simulink model "modello_completo_simulink2020"  (R2020a)
settings: Solver=VariableStepAuto  StartTime=0.0  StopTime=200  RelTol=1e-3
values from neighbouring files (symbols this model uses):
  a = 0.35    [data.m]    (also in geodetic2nedS.m = 6378137)
  a1 = rho * D^4 * alpha1    (= 0.000388302366464)    [data.m]
  a2 = -rho * D^3 * alpha2 * (1 - omega)    (= 0.0037030698432)    [data.m]
  AHRS_bias = [0 0 0]    [data.m]
  AHRS_sample_time = 1/50    (= 0.02)    [data.m]
  AHRS_var = ([1 1 2] * pi/180).^2    [data.m]
  alpha1 = 0.0113    [data.m]
  alpha2 = -0.0091    [data.m]
  c = son2(1)    [Sonar_id.m]    (also in data.m = 0.19)
  current = [seaCurrent; 0; 0; 0]    [data.m]
  D = 0.076    [data.m]
  dead_zone_limit = 31.5    [data.m]
  DVL_sample_t = 1/12    (= 0.0833333333333)    [data.m]
  DVL_var1 = 0.005^2    (= 2.5e-05)    [data.m]
  DVL_var2 = 0.015^2    (= 0.000225)    [data.m]
  DVL_var3 = 0.023^2    (= 0.000529)    [data.m]
  gps_sample_t = 1    [data.m]
  H = eye(3)    [data.m]    (also in navigation_data.m)
  IMU_sample_time = 1/100    (= 0.01)    [data.m]
  initial = []    [data.m]
  INSP = unicode2native(inspectionDirection)    [data.m]
  Ki_bodypos1 = 0    [parametri_PID.m]
  Ki_bodypos2 = 0    [parametri_PID.m]
  Ki_bodypos3 = 0    [parametri_PID.m]
  Ki_bodypos4 = 0    [parametri_PID.m]
  Ki_bodypos5 = 0    [parametri_PID.m]
  Ki_depth1 = 0    [parametri_PID.m]
  Ki_depth2 = 0    [parametri_PID.m]
  Ki_depth3 = 0    [parametri_PID.m]
  Ki_depth4 = 0    [parametri_PID.m]
  Ki_depth5 = 0    [parametri_PID.m]
  Ki_latvel1 = 0    [parametri_PID.m]
  Ki_latvel2 = 0    [parametri_PID.m]
  Ki_latvel3 = 0    [parametri_PID.m]
  Ki_latvel4 = 0    [parametri_PID.m]
  Ki_latvel5 = 0    [parametri_PID.m]
  Ki_P1 = 0    [parametri_PID.m]
  Ki_P2 = 0    [parametri_PID.m]
  Ki_P3 = 0    [parametri_PID.m]
  Ki_P4 = 0    [parametri_PID.m]
  Ki_P5 = 0    [parametri_PID.m]
  Ki_R1 = 0    [parametri_PID.m]
  Ki_R2 = 0    [parametri_PID.m]
  Ki_R3 = 0    [parametri_PID.m]
  Ki_R4 = 0    [parametri_PID.m]
  Ki_R5 = 0    [parametri_PID.m]
  Ki_rel_or1 = 0    [parametri_PID.m]
  Ki_rel_or2 = 0    [parametri_PID.m]
  Ki_rel_or3 = 0    [parametri_PID.m]
  Ki_rel_or4 = 0    [parametri_PID.m]
  Ki_rel_or5 = 0    [parametri_PID.m]
  Ki_reldist1 = 0    [parametri_PID.m]
  Ki_reldist2 = 0    [parametri_PID.m]
  Ki_reldist3 = 0    [parametri_PID.m]
  Ki_reldist4 = 0    [parametri_PID.m]
  Ki_reldist5 = 0    [parametri_PID.m]
  Ki_surge1 = 0    [parametri_PID.m]
  Ki_surge2 = 0    [parametri_PID.m]
  Ki_surge3 = 0    [parametri_PID.m]
  Ki_surge4 = 0    [parametri_PID.m]
  Ki_surge5 = 0    [parametri_PID.m]
  Ki_yaw1 = 0    [parametri_PID.m]
  Ki_yaw2 = 0    [parametri_PID.m]
  Ki_yaw3 = 0    [parametri_PID.m]
  Ki_yaw4 = 0    [parametri_PID.m]
  Ki_yaw5 = 0    [parametri_PID.m]
  Kp_bodypos1 = 0    [parametri_PID.m]
  Kp_bodypos2 = 2    [parametri_PID.m]
  Kp_bodypos3 = 2    [parametri_PID.m]
  Kp_bodypos4 = 2    [parametri_PID.m]
  Kp_bodypos5 = 2    [parametri_PID.m]
  Kp_depth1 = 0    [parametri_PID.m]
  Kp_depth2 = 2    [parametri_PID.m]
  Kp_depth3 = 2    [parametri_PID.m]
  Kp_depth4 = 2    [parametri_PID.m]
  Kp_depth5 = 2    [parametri_PID.m]
  Kp_latvel1 = 0    [parametri_PID.m]
  Kp_latvel2 = 2    [parametri_PID.m]
  Kp_latvel3 = 2    [parametri_PID.m]
  Kp_latvel4 = 2    [parametri_PID.m]
  Kp_latvel5 = 2    [parametri_PID.m]
  Kp_P1 = 0    [parametri_PID.m]
  Kp_P2 = 2    [parametri_PID.m]
  Kp_P3 = 2    [parametri_PID.m]
  Kp_P4 = 2    [parametri_PID.m]
  Kp_P5 = 2    [parametri_PID.m]
  Kp_R1 = 0    [parametri_PID.m]
  Kp_R2 = 2    [parametri_PID.m]
  Kp_R3 = 2    [parametri_PID.m]
  Kp_R4 = 2    [parametri_PID.m]
  Kp_R5 = 2    [parametri_PID.m]
  Kp_rel_or1 = 0    [parametri_PID.m]
  Kp_rel_or2 = 2    [parametri_PID.m]
  Kp_rel_or3 = 2    [parametri_PID.m]
  Kp_rel_or4 = 2    [parametri_PID.m]
  Kp_rel_or5 = 2    [parametri_PID.m]
  Kp_reldist1 = 0    [parametri_PID.m]
  Kp_reldist2 = 2    [parametri_PID.m]
  Kp_reldist3 = 2    [parametri_PID.m]
  Kp_reldist4 = 2    [parametri_PID.m]
  Kp_reldist5 = 2    [parametri_PID.m]
  Kp_surge1 = 0    [parametri_PID.m]
  Kp_surge2 = 2    [parametri_PID.m]
  Kp_surge3 = 2    [parametri_PID.m]
  Kp_surge4 = 2    [parametri_PID.m]
  Kp_surge5 = 2    [parametri_PID.m]
  Kp_yaw1 = 0.6*6    (= 3.6)    [parametri_PID.m]
  Kp_yaw2 = 2    [parametri_PID.m]
  Kp_yaw3 = 2    [parametri_PID.m]
  Kp_yaw4 = 2    [parametri_PID.m]
  Kp_yaw5 = 2    [parametri_PID.m]
  M = M_rb + M_a    [Masse.m]
  M_inv = inv(M)    [Masse.m]
  n_max = 340    [data.m]
  num_cycle = 5    [data.m]    (also in navigation_data.m)
  omega = 0.1    [data.m]
  plot_smpl = 0.1    [data.m]
  ps_sample_t = 0.02    [data.m]
  ps_var = (5000/3)^2    (= 2777777.77778)    [data.m]
  pylonCenter = [ 43.723046 ... (first row only)    [missionB.m]
  ... (+4 more)
undefined symbols (not defined in the file or in its folder): DiscIntNeverNeededParam, s_data
libraries: simulink x3
(part 2 of 5)

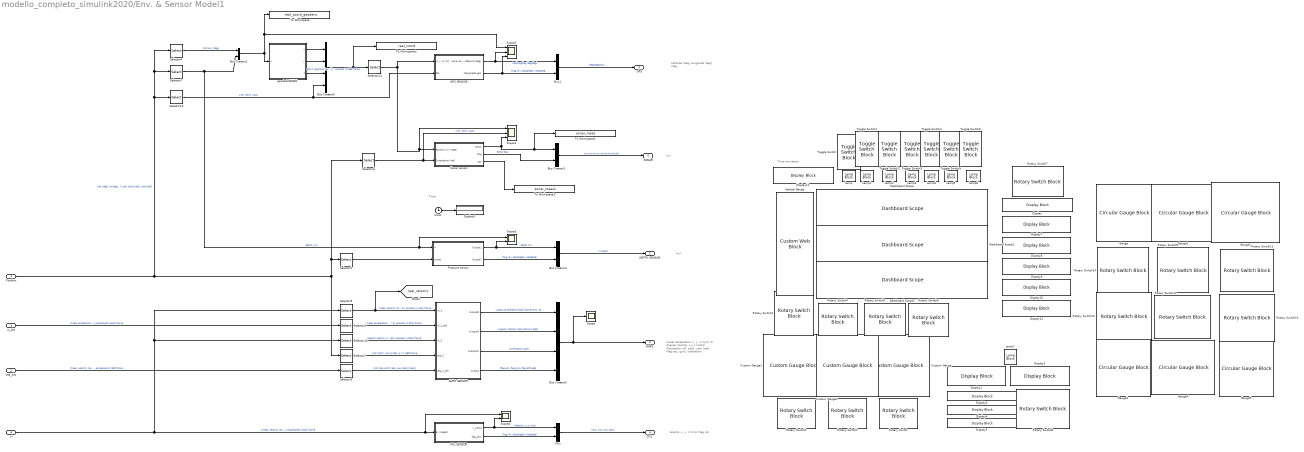
== system modello_completo_simulink2020/Env. & Sensor Model1 ==
  note: Time simulation
  note: Time
  note: (m)
  note: Velocity x, y, z (m/s)
      | Flag dvl
  note: Linear Acceleration x, y, z (m/s^2)
      | Angular Velocity x,y,z (rad/s)
      | Orientation roll, pitch, yaw (rad)
      | Flag acc, gyro, orientation
  note: (m)
  note: Latitude (deg)
      | Longitude (deg)
      | Flag
  Position : Inport
  eta_dot : Inport  Port=2
  ni_dot : Inport  Port=3
  ni : Inport  Port=4
  AHRS SENSOR : Subsystem
  Bus Creator2 : BusCreator  Inputs=2
  Bus Creator3 : BusCreator  Inputs=2
  Bus Creator4 : BusCreator  Inputs=2
  Bus Creator5 : BusCreator  Inputs=4
  Bus Creator6 : BusCreator  Inputs=4
  Clock : Clock
  Custom Gauge : CustomGaugeBlock  LabelPosition=Bottom  NeedleImage=data:image/svg+xml;base64,PD94bWwgdmVyc2lvbj0iMS4wIiBlbmNvZGluZz0idXRmLTgiPz4KPCEtLSBHZW5lcmF0b3I6IEFkb2JlIElsbHVzdHJhdG9yIDE5LjIuMSwgU1ZHIEV4cG9ydCBQbHVnLUluIC4gU1ZHIFZlcnNpb246IDYuMDAgQnVpbGQgMCkgIC0tPgo8c3ZnIHZlcnNpb249IjEuMSIgeG1sbnM9Imh0dHA6Ly93d3cudzMub3JnLzIwMDAvc3ZnIiB4bWxuczp4bGluaz0iaHR0cDovL3d3dy53My5vcmcvMTk5OS94bGluayIgeD0iMHB4IiB5PSIwcHgiCgkgdmlld0JveD0iMCAwIDIwMCA1MCIgc3R5bGU9ImVuYWJsZS1iYWNrZ3JvdW5kOm5ldyAw ...(+9940 chars)  NeedleXPos=0.4166541406625117  NeedleYPos=0.48689867826277666  NeedleHeight=0.08073723570250356  NeedleWidth=0.1330086340281622  NeedleInitialRotation=-59.94322499147643  BackgroundImage=data:image/svg+xml;base64,PD94bWwgdmVyc2lvbj0iMS4wIiBlbmNvZGluZz0iVVRGLTgiIHN0YW5kYWxvbmU9Im5vIj8+CjwhLS0gR2VuZXJhdG9yOiBBZG9iZSBJbGx1c3RyYXRvciAxOS4yLjEsIFNWRyBFeHBvcnQgUGx1Zy1JbiAuIFNWRyBWZXJzaW9uOiA2LjAwIEJ1aWxkIDApICAtLT4KCjxzdmcKICAgeG1sbnM6ZGM9Imh0dHA6Ly9wdXJsLm9yZy9kYy9lbGVtZW50cy8xLjEvIgogICB4bWxuczpjYz0iaHR0cDovL2NyZWF0aXZlY29tbW9ucy5vcmcvbnMjIgogICB4bWxuczpyZGY9Imh0dHA6Ly93d3cudzMub3JnLzE5OTkvMDIvMjItcmRmLXN5bnRh ...(+9660 chars)  GaugeMin=-1  GaugeMax=1  GaugeArcDefined=true  GaugeArcRadius=0.09453995649289303  GaugeArcStrokeWidth=0.027647132727189508  GaugeArcRotation=240.5385250290321  GaugeArcRatio=0.8333333333333  GaugeArcTransparency=0  ValueArcColor=#1759b0  GaugeTickColor=#faf5c8  ScaleColorsJSON=[]  fixedAspectRatio=on  IsLinearGauge=false  GaugeTrackLeft=0.35  GaugeTrackTop=0.35  GaugeTrackHeight=0.1  GaugeTrackWidth=0.3  GaugeTrackRotation=0  ScaleMin=-1
  Custom Gauge1 : CustomGaugeBlock  LabelPosition=Bottom  NeedleImage=data:image/svg+xml;base64,PD94bWwgdmVyc2lvbj0iMS4wIiBlbmNvZGluZz0idXRmLTgiPz4KPCEtLSBHZW5lcmF0b3I6IEFkb2JlIElsbHVzdHJhdG9yIDE5LjIuMSwgU1ZHIEV4cG9ydCBQbHVnLUluIC4gU1ZHIFZlcnNpb246IDYuMDAgQnVpbGQgMCkgIC0tPgo8c3ZnIHZlcnNpb249IjEuMSIgeG1sbnM9Imh0dHA6Ly93d3cudzMub3JnLzIwMDAvc3ZnIiB4bWxuczp4bGluaz0iaHR0cDovL3d3dy53My5vcmcvMTk5OS94bGluayIgeD0iMHB4IiB5PSIwcHgiCgkgdmlld0JveD0iMCAwIDIwMCA1MCIgc3R5bGU9ImVuYWJsZS1iYWNrZ3JvdW5kOm5ldyAw ...(+9940 chars)  NeedleXPos=0.4141461298017858  NeedleYPos=0.4865044384352907  NeedleHeight=0.08316674888547909  NeedleWidth=0.13701107759722064  NeedleInitialRotation=-59.94322499147643  BackgroundImage=data:image/svg+xml;base64,PD94bWwgdmVyc2lvbj0iMS4wIiBlbmNvZGluZz0iVVRGLTgiIHN0YW5kYWxvbmU9Im5vIj8+CjwhLS0gR2VuZXJhdG9yOiBBZG9iZSBJbGx1c3RyYXRvciAxOS4yLjEsIFNWRyBFeHBvcnQgUGx1Zy1JbiAuIFNWRyBWZXJzaW9uOiA2LjAwIEJ1aWxkIDApICAtLT4KCjxzdmcKICAgeG1sbnM6ZGM9Imh0dHA6Ly9wdXJsLm9yZy9kYy9lbGVtZW50cy8xLjEvIgogICB4bWxuczpjYz0iaHR0cDovL2NyZWF0aXZlY29tbW9ucy5vcmcvbnMjIgogICB4bWxuczpyZGY9Imh0dHA6Ly93d3cudzMub3JnLzE5OTkvMDIvMjItcmRmLXN5bnRh ...(+9660 chars)  GaugeMin=-1  GaugeMax=1  GaugeArcDefined=true  GaugeArcRadius=0.09738481572815044  GaugeArcStrokeWidth=0.028479079385354485  GaugeArcRotation=240.5385250290321  GaugeArcRatio=0.8333333333333  GaugeArcTransparency=0  ValueArcColor=#1759b0  GaugeTickColor=#faf5c8  ScaleColorsJSON=[]  fixedAspectRatio=on  IsLinearGauge=false  GaugeTrackLeft=0.35  GaugeTrackTop=0.35  GaugeTrackHeight=0.1  GaugeTrackWidth=0.3  GaugeTrackRotation=0  ScaleMin=-1
  Custom Gauge2 : CustomGaugeBlock  LabelPosition=Bottom  NeedleImage=data:image/svg+xml;base64,PD94bWwgdmVyc2lvbj0iMS4wIiBlbmNvZGluZz0idXRmLTgiPz4KPCEtLSBHZW5lcmF0b3I6IEFkb2JlIElsbHVzdHJhdG9yIDE5LjIuMSwgU1ZHIEV4cG9ydCBQbHVnLUluIC4gU1ZHIFZlcnNpb246IDYuMDAgQnVpbGQgMCkgIC0tPgo8c3ZnIHZlcnNpb249IjEuMSIgeG1sbnM9Imh0dHA6Ly93d3cudzMub3JnLzIwMDAvc3ZnIiB4bWxuczp4bGluaz0iaHR0cDovL3d3dy53My5vcmcvMTk5OS94bGluayIgeD0iMHB4IiB5PSIwcHgiCgkgdmlld0JveD0iMCAwIDIwMCA1MCIgc3R5bGU9ImVuYWJsZS1iYWNrZ3JvdW5kOm5ldyAw ...(+9940 chars)  NeedleXPos=0.4166541406625117  NeedleYPos=0.48689867826277666  NeedleHeight=0.08073723570250356  NeedleWidth=0.1330086340281622  NeedleInitialRotation=-59.94322499147643  BackgroundImage=data:image/svg+xml;base64,PD94bWwgdmVyc2lvbj0iMS4wIiBlbmNvZGluZz0iVVRGLTgiIHN0YW5kYWxvbmU9Im5vIj8+CjwhLS0gR2VuZXJhdG9yOiBBZG9iZSBJbGx1c3RyYXRvciAxOS4yLjEsIFNWRyBFeHBvcnQgUGx1Zy1JbiAuIFNWRyBWZXJzaW9uOiA2LjAwIEJ1aWxkIDApICAtLT4KCjxzdmcKICAgeG1sbnM6ZGM9Imh0dHA6Ly9wdXJsLm9yZy9kYy9lbGVtZW50cy8xLjEvIgogICB4bWxuczpjYz0iaHR0cDovL2NyZWF0aXZlY29tbW9ucy5vcmcvbnMjIgogICB4bWxuczpyZGY9Imh0dHA6Ly93d3cudzMub3JnLzE5OTkvMDIvMjItcmRmLXN5bnRh ...(+9660 chars)  GaugeMin=-1  GaugeMax=1  GaugeArcDefined=true  GaugeArcRadius=0.09453995649289303  GaugeArcStrokeWidth=0.027647132727189508  GaugeArcRotation=240.5385250290321  GaugeArcRatio=0.8333333333333  GaugeArcTransparency=0  ValueArcColor=#1759b0  GaugeTickColor=#faf5c8  ScaleColorsJSON=[]  fixedAspectRatio=on  IsLinearGauge=false  GaugeTrackLeft=0.35  GaugeTrackTop=0.35  GaugeTrackHeight=0.1  GaugeTrackWidth=0.3  GaugeTrackRotation=0  ScaleMin=-1
  DVL SENSOR : Subsystem
  Dashboard Scope : DashboardScope  Ymin=-12  Ymax=12  LegendPosition=Right
  Dashboard Scope1 : DashboardScope  Ymin=-1  Ymax=1  LegendPosition=Right
  Dashboard Scope2 : DashboardScope  Ymin=-2  Ymax=2  LegendPosition=Right
  Display : DisplayBlock  LabelPosition=Hide  Format=Custom  Transparency=1  FormatString=Sonar flag: %d %d %d %d %d
  Display1 : DisplayBlock  LabelPosition=Hide  Format=Custom  Transparency=1  FormatString=Lat: %f °
  Display{8..11} (4 alike) : DisplayBlock  Format=short  Transparency=1
  Display12 : DisplayBlock  LabelPosition=Hide  Format=Custom  Transparency=1  FormatString=%.1f s
  Display2 : DisplayBlock  LabelPosition=Hide  Format=Custom  Transparency=1  FormatString=Lon: %f °
  Display3 : DisplayBlock  LabelPosition=Hide  Format=Custom  Transparency=1  FormatString=X NED: %.3f m
  Display4 : DisplayBlock  LabelPosition=Hide  Format=Custom  Transparency=1  FormatString=Y NED: %.3f m
  Display5 : DisplayBlock  LabelPosition=Hide  Format=Custom  Transparency=1  FormatString=Z NED: %.3f m
  Display6 : Display
  Display7 : DisplayBlock  Format=short  Transparency=1  FormatString=%d m
  GPS SENSOR : Subsystem
  Gauge : CircularGaugeBlock  ScaleMin=-25  ScaleMax=25
  Gauge1 : CircularGaugeBlock  ScaleMin=-25  ScaleMax=25
  Gauge2 : CircularGaugeBlock  ScaleMin=-25  ScaleMax=25
  Gauge3 : CircularGaugeBlock  LabelPosition=Bottom  ScaleMin=-45  ScaleMax=45
  Gauge4 : CircularGaugeBlock  LabelPosition=Bottom  ScaleMin=-45  ScaleMax=45
  Gauge5 : CircularGaugeBlock  LabelPosition=Bottom  ScaleMin=-45  ScaleMax=45
  Lamp{,1..7} (8 alike) : LampBlock  LabelPosition=Hide
  Mux : Mux  Inputs=2
  Mux1 : Mux  Inputs=2
  Pressure sensor : Subsystem
  Rotary Switch{,1..8} (9 alike) : RotarySwitchBlock  LabelPosition=Bottom
      settings: Values={{'Off', 'On', '50%', '200%'}, [0 1 0.5 2]}
  Rotary Switch{9..14} (6 alike) : RotarySwitchBlock
  Scope : Scope
  Scope1 : Scope  NumInputPorts=3
  Scope2 : Scope  NumInputPorts=3
  Scope3 : Scope  NumInputPorts=2
  Scope4 : Scope  NumInputPorts=2
  Selector{1..3,6,10,12} (6 alike) : Selector  InputPortWidth=6  IndexOptions=Index vector (dialog)  Indices=[4 5 6]  OutputSizes=1
  Selector14 : Selector  InputPortWidth=6  IndexOptions=Index vector (dialog)  Indices=[1 2 3]  OutputSizes=1
  Selector4 : Selector  InputPortWidth=6  IndexOptions=Index vector (dialog)  Indices=[1 2]  OutputSizes=1
  Selector5 : Selector  InputPortWidth=6  IndexOptions=Index vector (dialog)  Indices=[1 2 3]  OutputSizes=1
  Selector7 : Selector  InputPortWidth=6  IndexOptions=Index vector (dialog)  Indices=[3]  OutputSizes=1
  Selector9 : Selector  InputPortWidth=6  IndexOptions=Index vector (dialog)  Indices=[1 2 3]  OutputSizes=1
  Sonar sensor : Subsystem
  To Workspace : ToWorkspace  VariableName=real_coord_geodetic  SampleTime=-1
  To Workspace1 : ToWorkspace  VariableName=sonar_meas  SampleTime=plot_smpl
  To Workspace2 : ToWorkspace  VariableName=real_coord  SampleTime=plot_smpl
  To Workspace3 : ToWorkspace  VariableName=sonar_meas1  SampleTime=plot_smpl
  Toggle Switch{,2,4,6} (4 alike) : ToggleSwitchBlock  LabelPosition=Bottom
      settings: Values={{'Off', 'On'}, [0 1]}
  Toggle Switch1 : ToggleSwitchBlock
      settings: Values={{'Off', 'On'}, [1 0]}
  Toggle Switch3 : ToggleSwitchBlock
      settings: Values={{'Off', 'On'}, [0 1]}
  Toggle Switch5 : ToggleSwitchBlock
      settings: Values={{'Off', 'On'}, [0 1]}
  Vertical Gauge : CustomWebBlock  ShowInitialText=on  Configuration="{\"components\":[{\"name\":\"LinearScaleComponent\",\"settings\":{\"bounds\":{\"max\":40,\"min\":0,\"tickInterval\":\"auto\"},\"labelColor\":[250,245,199],\"labelFont\":{\"font\":\"Arial\",\"fontSize\":12},\"labelTransparency\":1,\"needleImage\":{\"size\":[21,75],\"src\":\"data:image\\/svg+xml;base64,PHN2ZyB4bWxucz0iaHR0cDovL3d3dy53My5vcmcvMjAwMC9zdmciIHhtbG5zOnhsaW5rPSJodHRwOi8vd3d3LnczLm9yZy8xOTk5L3hsaW5rIiB2aWV3Qm94PSIwIDAgMjEgNzUiPjxkZWZzPjxzdHlsZT4uY2xzLTF7ZmlsbDpub25lO30uY2xzLTJ7aXNvbGF0aW9uOmlzb2xhdGU7fS5jbHMtM3tjbGlwLXBhdGg6dXJsKCNjbGlwLXBhdGgpO30uY2xzLTR7b3BhY2l0eTowLjM7bWl4LWJsZW5kLW1vZGU6bXVsdGlwbHk7fS5jbHMtNXtmaWxsOiNlYjI2Mjk7fTwvc3R5bGU+PGNsaXBQYXRoIGlkPSJjbGlwLXBhdGgiIHRyYW5zZm9y ...(+1928 chars)\",\"srcOrientation\":\"horizontal\"},\"needleOffset\":[-0.01094391244870041,0],\"needleSize\":{\"height\":0.11960078534031414,\"width\":0.7589285714285714},\"position\":[0.015887605042016806,0.06986607142857143,0.8,0.9641544117647058],\"scaleColorSize\":0.24,\"scaleColors\":[],\"scaleColorsSize\":0.2,\"tickColor\":[250,245,200],\"tickTransparency\":1,\"valueBarColor\":[23,89,176],\"valueBarSize\":0.23,\"valueBarTransparency\":1}},{\"name\":\"BackgroundImageComponent\",\"settings\":{\"image\":{\"size\":[380,101],\"src\":\"data:image\\/svg+xml;base64,PHN2ZyB4bWxucz0iaHR0cDovL3d3dy53My5vcmcvMjAwMC9zdmciIHhtbG5zOnhsaW5rPSJodHRwOi8vd3d3LnczLm9yZy8xOTk5L3hsaW5rIiB2aWV3Qm94PSIwIDAgMzgwIDEwMSI+PGRlZnM+PHN0eWxlPi5jbHMtMXtmaWxsOnVybCgjbGluZWFyLWdyYWRpZW50KTt9LmNscy0ye2ZpbGw6dXJsKCNsaW5lYXItZ3JhZGllbnQtMik7fS5jbHMtM3tmaWxsOnVybCgjbGluZWFyLWdyYWRpZW50LTMpO308L3N0eWxlPjxsaW5lYXJHcmFkaWVudCBpZD0ibGluZWFyLWdyYWRpZW50IiB5MT0iNTAuNSIgeDI9IjM5OS4yOCIgeTI9IjUw ...(+2216 chars)\",\"srcOrientation\":\"horizontal\"},\"position\":[0,0,1,1],\"scaleMode\":\"0\"}}],\"settings\":{\"BindingType\":\"signal\",\"fixedAspectRatio\":\"on\",\"orientation\":\"vertical\"},\"type\":\"LinearGauge\"}"
  geodetic2NED1 : MATLAB Function  TreatAsAtomicUnit=on
  GPS : Outport
  DEPTH SENSOR : Outport  Port=2
  AHRS : Outport  Port=3
  "DVL " : Outport  Port=4
  SONAR : Outport  Port=5
  tag scope: real_velocity=global
  wires:
  Pressure sensor/1(Output1) -> Bus Creator4/1, Scope3/2  "depth (m)"
  AHRS SENSOR/1(Output8) -> Bus Creator5/1  "Linear Acceleration body frame [m/s^2]"
  Mux1/1 -> GPS/1  "(deg/deg/bool)"
  AHRS SENSOR/3(Output10) -> Bus Creator5/3  "Orientation [rad]"
  Bus Creator6/1 -> To Workspace2/1, Selector14/1  "eta = [position (3x1),  \t  orientation (3x1)], \t  express in NED frame."
  Selector14/1 -> GPS SENSOR/1("[x, y, z] [m]"), Scope1/1, Sonar sensor/1(Position (m) (NED))
  GPS SENSOR/1(Lat e Lon Measure [deg]) -> Scope2/2, Mux1/1  "Lat/long/flag (deg/deg)"
  Selector7/1 -> Bus Creator2/2, Scope3/1, Pressure sensor/1(h)  "depth, [m]"
  geodetic2NED1/3(z) -> Bus Creator6/3
  Selector2/1 -> AHRS SENSOR/4(eta_2)  "[roll  pitch  yaw] [rad], w.r.t. NED frame"
  Bus Creator5/1 -> Scope/1, AHRS/1
  AHRS SENSOR/2(Output9) -> Bus Creator5/2  "Angular Velocity body frame [rad/s]"
  ni/1 -> DVL SENSOR/1(By model2), Scope4/1, Selector10/1, Selector5/1  "[linear velocity (3x1),angular velocity (3x1)], expressed in body frame."
  Selector6/1 -> Sonar sensor/2(Orientation (rad)), Scope1/2  "[roll  pitch  yaw]"
  AHRS SENSOR/4(Output) -> Bus Creator5/4  "[flag acc, flag gyro, flag attitude]"
  GPS SENSOR/2(Flag enable gps) -> Scope2/3, Mux1/2  "Flag (0->disabled/1->Enabled)"
  Selector10/1 -> AHRS SENSOR/3(ni_2)  "angular velocity [rad/s], express in body frame"
  eta_dot/1 -> Selector3/1  "[linear velocity (3x1), roll rate, pitch rate, yaw rate] , expressed in NED frame."
  Selector9/1 -> AHRS SENSOR/2(ni_1_dot)  "linear acceleration [m/s^2], express in body frame"
  Pressure sensor/2(Output7) -> Bus Creator4/2  "Flag (0->disabled/1->Enabled)"
  Selector4/1 -> Bus Creator2/1  "[lat lon], [deg]"
  DVL SENSOR/2(flag_DVL) -> Mux/2  "Flag (0->disabled/1->Enabled)"
  Mux/1 -> "DVL "/1  "(m/s, m/s, m/s, bool)"
  geodetic2NED1/1(x) -> Bus Creator6/1
  geodetic2NED1/2(y) -> Bus Creator6/2
  Selector3/1 -> AHRS SENSOR/5(eta_2_dot)  "[roll rate, pitch rate, yaw rate] [rad/s]"
  Position/1 -> Selector2/1, Selector1/1, Selector6/1, Selector4/1, Selector7/1, Selector12/1  "[lat (deg), lon(deg), depth(m), roll (rad), pitch(rad), yaw(rad)]"
  Bus Creator4/1 -> DEPTH SENSOR/1  "(m,bool)"
  Selector5/1 -> [real_velocity], AHRS SENSOR/1(ni_1)  "linear velocity [m/s], express in body frame"
  ni_dot/1 -> Selector9/1  "[linear acceleration (3x1), angular acceleration (3x1)], expressed in body frame."
  Bus Creator2/1 -> To Workspace/1, Scope2/1, geodetic2NED1/1(u)
  DVL SENSOR/1(v_sens1) -> Scope4/2, Mux/1  "Velocity x,y,z (m/s)"
  Bus Creator3/1 -> SONAR/1  "(m,m,m,m,m, int,int,int,int,int)"
  Selector12/1 -> Bus Creator6/4, GPS SENSOR/2(eta)  "[roll  pitch  yaw]"
  Selector1/1 -> Pressure sensor/2(orient)
  Sonar sensor/1(Sonar) -> To Workspace1/1, Bus Creator3/1, Scope1/3
  Sonar sensor/3(Son) -> To Workspace3/1
  Sonar sensor/2(Flag) -> Bus Creator3/2  "Sonar flag"
  Clock/1 -> Display6/1
